simulink model "geometric_control_improved_apf"  (R2025a)
settings: Solver=VariableStepAuto  StartTime=0.0  StopTime=50  RelTol=1e-3
values from neighbouring files (symbols this model uses):
  Ib = diag([1.2416 1.2416 2*1.2416])    [main_geometric_control_improved_apf.m]
  K_a = 1.0    (= 1)    [main_geometric_control_improved_apf.m]
  K_r = 0.5    [main_geometric_control_improved_apf.m]
  K_v = 0.1    [main_geometric_control_improved_apf.m]
  lin_vel_0 = [0; 0; 0]    [main_geometric_control_improved_apf.m]
  mass = 1.2    [main_geometric_control_improved_apf.m]
  obstacles_points = [obstacles_points, points]    [main_geometric_control_improved_apf.m]
  pos_0 = [x0 y0 z0]    [main_geometric_control_improved_apf.m]
  pos_goal = [xf yf zf]    [main_geometric_control_improved_apf.m]
  psif = 0    [main_geometric_control_improved_apf.m]
  rho_0 = 2.0    (= 2)    [main_geometric_control_improved_apf.m]
  Ts = 0.01    [main_geometric_control_improved_apf.m]
  w_bb_0 = [0; 0; 0]    [main_geometric_control_improved_apf.m]
undefined symbols (not defined in the file or in its folder): DiscIntNeverNeededParam
libraries: uavsimlib x3, robotcorelib x2, eeGeneralControl x1
settings Model: Creator=emman  LastModifiedBy=emman

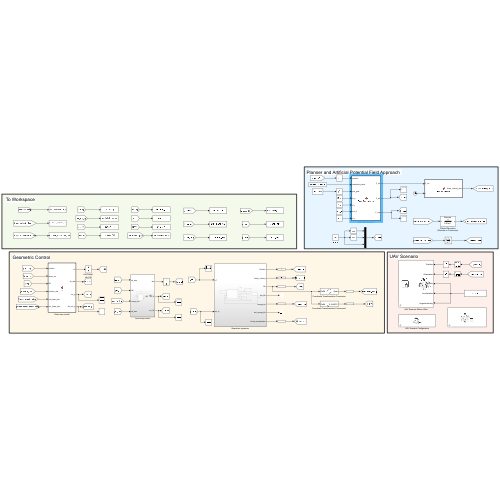
[thumbnail: Simulink's stored preview of the top-level diagram]
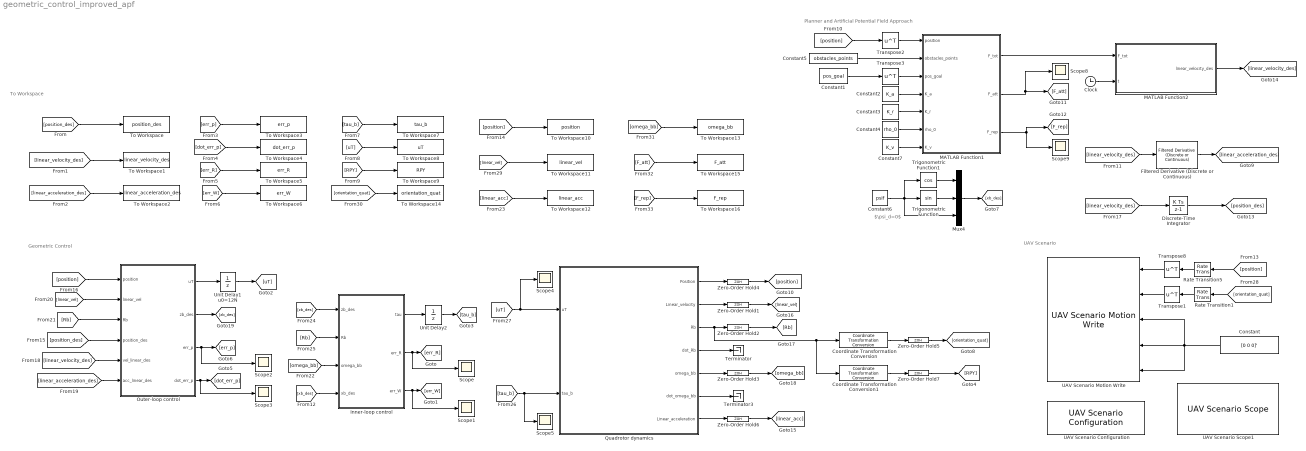
== system geometric_control_improved_apf ==
  note: Planner and Artificial Potential Field Approach
  note: Geometric Control
  note: UAV Scenario
  note: $\psi_d=0$
  note: To Workspace
  Clock : Clock
  Constant : Constant  Value=[0 0 0]'
  Constant1 : Constant  Value=pos_goal
  Constant2 : Constant  Value=K_a
  Constant3 : Constant  Value=K_r
  Constant4 : Constant  Value=rho_0
  Constant5 : Constant  Value=obstacles_points
  Constant6 : Constant  Value=psif
  Constant7 : Constant  Value=K_v
  Coordinate Transformation Conversion : robotcorelib/Coordinate Transformation Conversion  InputRepresentation=Rotation Matrix  InputEulerSequence=ZYX  ShowTrVecInputPort=on  OutputRepresentation=Quaternion  OutputEulerSequence=ZYX  ShowTrVecOutputPort=on  SimulateUsing=Interpreted execution
  Coordinate Transformation Conversion1 : robotcorelib/Coordinate Transformation Conversion  InputRepresentation=Rotation Matrix  InputEulerSequence=ZYX  ShowTrVecInputPort=on  OutputRepresentation=Euler Angles  OutputEulerSequence=ZYX  ShowTrVecOutputPort=on  SimulateUsing=Interpreted execution
  Discrete-Time Integrator : DiscreteIntegrator  InitialCondition=pos_0  SampleTime=Ts  ICPrevOutput=DiscIntNeverNeededParam  ICPrevScaledInput=DiscIntNeverNeededParam
  Filtered Derivative (Discrete or Continuous) : eeGeneralControl/Filtered Derivative (Discrete or Continuous)  K=1  T=Ts  B=inf  A=-inf  minRatio=10  init_option=Inherited from block input  x0=0  Ts=-1
      settings: LibrarySourceBlock=|
      | ee_sl_lib/General Control/Filtered Derivative
      | (Discrete or Continuous)
  Inner-loop control : Subsystem
  MATLAB Function1 : MATLAB Function  TreatAsAtomicUnit=on
  MATLAB Function2 : MATLAB Function  TreatAsAtomicUnit=on
  Mux4 : Mux  Inputs=3
  Outer-loop control : MATLAB Function  TreatAsAtomicUnit=on
  Quadrotor dynamics : Subsystem
  Rate Transition1 : RateTransition  OutPortSampleTime=Ts
  Rate Transition5 : RateTransition  OutPortSampleTime=Ts
  Scope{,1..5,8..9} (8 alike) : Scope
      Scope settings: ActiveDisplayYMinimum=-3.1E-6  ActiveDisplayYMaximum=3.1E-6
      Scope1 settings: ActiveDisplayYMinimum=-1.2E-5  ActiveDisplayYMaximum=1.2E-5
      Scope2 settings: ActiveDisplayYMinimum=-1E-5  ActiveDisplayYMaximum=2E-6  DataLoggingVariableName=ScopeData6
      Scope3 settings: ActiveDisplayYMinimum=-0.00022  ActiveDisplayYMaximum=5E-5  DataLoggingVariableName=ScopeData3
      Scope4 settings: ActiveDisplayYMinimum=11.66748  ActiveDisplayYMaximum=12.03695  DataLoggingVariableName=ScopeData4
      Scope5 settings: ActiveDisplayYMinimum=-0.02035  ActiveDisplayYMaximum=0.02035  DataLoggingVariableName=ScopeData5
      Scope8 settings: ActiveDisplayYMinimum=-10.489441161556352  ActiveDisplayYMaximum=10.433654100091561  DataLoggingVariableName=ScopeData8
      Scope9 settings: ActiveDisplayYMinimum=-1  ActiveDisplayYMaximum=1  DataLoggingVariableName=ScopeData9
  Terminator : Terminator
  Terminator3 : Terminator
  To Workspace : ToWorkspace  VariableName=position_des  SaveFormat=Timeseries  SampleTime=-1
  To Workspace1 : ToWorkspace  VariableName=linear_velocity_des  SaveFormat=Timeseries  SampleTime=-1
  To Workspace10 : ToWorkspace  VariableName=position  SaveFormat=Timeseries  SampleTime=-1
  To Workspace11 : ToWorkspace  VariableName=linear_vel  SaveFormat=Timeseries  SampleTime=-1
  To Workspace12 : ToWorkspace  VariableName=linear_acc  SaveFormat=Timeseries  SampleTime=-1
  To Workspace13 : ToWorkspace  VariableName=omega_bb  SaveFormat=Timeseries  SampleTime=-1
  To Workspace14 : ToWorkspace  VariableName=orientation_quat  SaveFormat=Timeseries  SampleTime=-1
  To Workspace15 : ToWorkspace  VariableName=F_att  SaveFormat=Timeseries  SampleTime=-1
  To Workspace16 : ToWorkspace  VariableName=F_rep  SaveFormat=Timeseries  SampleTime=-1
  To Workspace2 : ToWorkspace  VariableName=linear_acceleration_des  SaveFormat=Timeseries  SampleTime=-1
  To Workspace3 : ToWorkspace  VariableName=err_p  SaveFormat=Timeseries  SampleTime=-1
  To Workspace4 : ToWorkspace  VariableName=dot_err_p  SaveFormat=Timeseries  SampleTime=-1
  To Workspace5 : ToWorkspace  VariableName=err_R  SaveFormat=Timeseries  SampleTime=-1
  To Workspace6 : ToWorkspace  VariableName=err_W  SaveFormat=Timeseries  SampleTime=-1
  To Workspace7 : ToWorkspace  VariableName=tau_b  SaveFormat=Timeseries  SampleTime=-1
  To Workspace8 : ToWorkspace  VariableName=uT  SaveFormat=Timeseries  SampleTime=-1
  To Workspace9 : ToWorkspace  VariableName=RPY  SaveFormat=Timeseries  SampleTime=-1
  Transpose{1..3,8} (4 alike) : Math  Operator=transpose
  Trigonometric Function : Trigonometry
  Trigonometric Function1 : Trigonometry  Operator=cos
  UAV Scenario Configuration : uavsimlib/UAV Scenario Configuration  Priority=-1  UAVScenarioObject=Scenario  SampleTime=Ts  UpdateParam=false  SensorMotionBusName='SensorMotionBus'  PlatformMotionBusName='PlatformMotionBus'  ScenarioMotionBusName='ScenarioMotionBus'  ScenarioMotionSignalName='ScenarioMotions'
  UAV Scenario Motion Write : uavsimlib/UAV Scenario Motion Write  Priority=0  PlatName='UAV'  ReferenceFrame=NED
  UAV Scenario Scope1 : uavsimlib/UAV Scenario Scope  Priority=1  SensorNameTable={}  SampleTime=Ts
  Unit Delay1 u0=12N : UnitDelay  InitialCondition=12  SampleTime=Ts
  Unit Delay2 : UnitDelay  InitialCondition=[0 0 0]  SampleTime=Ts
  Zero-Order Hold{1..7} (7 alike) : ZeroOrderHold  SampleTime=Ts
  wires:
  [linear_velocity_des] -> To Workspace1/1
  Zero-Order Hold3/1 -> [omega_bb]
  [tau_b] -> To Workspace7/1
  [err_R] -> To Workspace5/1
  Coordinate Transformation Conversion1/1 -> Zero-Order Hold7/1
  Coordinate Transformation Conversion/1 -> Zero-Order Hold5/1
  [position_des] -> To Workspace/1
  Quadrotor dynamics/3(Rb) -> Zero-Order Hold2/1, Coordinate Transformation Conversion1/1, Coordinate Transformation Conversion/1
  [err_W] -> To Workspace6/1
  Quadrotor dynamics/6(dot_omega_bb) -> Terminator3/1
  Outer-loop control/3(err_p) -> [err_p], Scope2/1
  Quadrotor dynamics/5(omega_bb) -> Zero-Order Hold3/1
  Outer-loop control/4(dot_err_p) -> [dot_err_p], Scope3/1
  [linear_acceleration_des] -> To Workspace2/1
  Quadrotor dynamics/2(Linear_velocity) -> Zero-Order Hold1/1
  Outer-loop control/1(uT) -> Unit Delay1 u0=12N/1
  Inner-loop control/2(err_R) -> [err_R], Scope/1
  Inner-loop control/3(err_W) -> Scope1/1, [err_W]
  Quadrotor dynamics/4(dot_Rb) -> Terminator/1
  [dot_err_p] -> To Workspace4/1
  [uT] -> To Workspace8/1
  [RPY] -> To Workspace9/1
  Inner-loop control/1(tau) -> Unit Delay2/1
  [err_p] -> To Workspace3/1
  Quadrotor dynamics/1(Position) -> Zero-Order Hold4/1
  Constant2/1 -> MATLAB Function1/4(K_a)
  Constant3/1 -> MATLAB Function1/5(K_r)
  Constant4/1 -> MATLAB Function1/6(rho_0)
  MATLAB Function1/1(F_tot) -> MATLAB Function2/1(F_tot)
  Clock/1 -> MATLAB Function2/2(t)
  MATLAB Function1/2(F_att) -> Scope8/1, [F_att]
  Trigonometric Function1/1 -> Mux4/1
  Mux4/1 -> [xb_des]
  Constant6/1 -> Mux4/3, Trigonometric Function/1, Trigonometric Function1/1
  Trigonometric Function/1 -> Mux4/2
  MATLAB Function2/1(linear_velocity_des) -> [linear_velocity_des]
  [linear_velocity_des] -> Filtered Derivative (Discrete or Continuous)/1
  Filtered Derivative (Discrete or Continuous)/1 -> [linear_acceleration_des]
  [xb_des] -> Inner-loop control/4(xb_des)
  [linear_velocity_des] -> Discrete-Time Integrator/1
  Zero-Order Hold1/1 -> [linear_vel]
  Zero-Order Hold2/1 -> [Rb]
  Zero-Order Hold4/1 -> [position]
  Constant/1 -> UAV Scenario Motion Write/5, UAV Scenario Motion Write/3, UAV Scenario Motion Write/4
  Discrete-Time Integrator/1 -> [position_des]
  Constant5/1 -> MATLAB Function1/2(obstacles_points)
  [position_des] -> Outer-loop control/4(position_des)
  [linear_velocity_des] -> Outer-loop control/5(vel_linear_des)
  [linear_acceleration_des] -> Outer-loop control/6(acc_linear_des)
  Rate Transition5/1 -> Transpose8/1
  [position] -> Rate Transition5/1
  Zero-Order Hold5/1 -> [orientation_quat]
  Quadrotor dynamics/7(Linear_acceleration) -> Zero-Order Hold6/1
  Zero-Order Hold6/1 -> [linear_acc]
  Zero-Order Hold7/1 -> [RPY]
  Outer-loop control/2(zb_des) -> [zb_des]
  [zb_des] -> Inner-loop control/1(zb_des)
  [omega_bb] -> Inner-loop control/3(omega_bb)
  [Rb] -> Inner-loop control/2(Rb)
  Unit Delay2/1 -> [tau_b]
  [tau_b] -> Scope5/1, Quadrotor dynamics/2(tau_b)
  Unit Delay1 u0=12N/1 -> [uT]
  [uT] -> Scope4/1, Quadrotor dynamics/1(uT)
  [position] -> Outer-loop control/1(position)
  [linear_vel] -> Outer-loop control/2(linear_vel)
  [Rb] -> Outer-loop control/3(Rb)
  Transpose8/1 -> UAV Scenario Motion Write/1
  Rate Transition1/1 -> Transpose1/1
  Transpose1/1 -> UAV Scenario Motion Write/2
  [orientation_quat] -> Rate Transition1/1
  [position] -> To Workspace10/1
  [linear_acc] -> To Workspace12/1
  [linear_vel] -> To Workspace11/1
  [omega_bb] -> To Workspace13/1
  [orientation_quat] -> To Workspace14/1
  [F_rep] -> To Workspace16/1
  [F_att] -> To Workspace15/1
  [position] -> Transpose2/1
  Transpose2/1 -> MATLAB Function1/1(position)
  Constant1/1 -> Transpose3/1
  MATLAB Function1/3(F_rep) -> Scope9/1, [F_rep]
  Transpose3/1 -> MATLAB Function1/3(pos_goal)
  Constant7/1 -> MATLAB Function1/7(K_v)

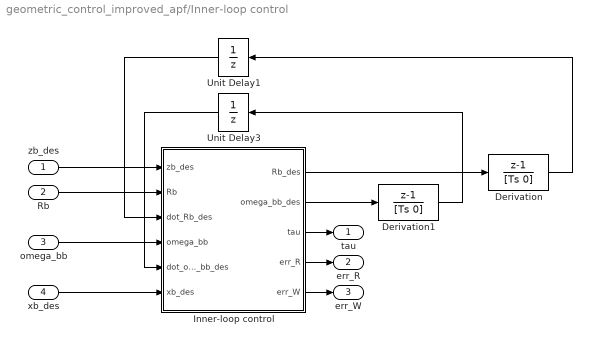
== system geometric_control_improved_apf/Inner-loop control ==
  zb_des : Inport
  Rb : Inport  Port=2
  omega_bb : Inport  Port=3
  xb_des : Inport  Port=4
  Derivation : DiscreteTransferFcn  Numerator=[1 -1]  Denominator=[Ts 0]  InitialStates=[1 0 0;0 1 0;0 0 1]  SampleTime=Ts
  Derivation1 : DiscreteTransferFcn  Numerator=[1 -1]  Denominator=[Ts 0]  InitialStates=[0 0 0]  SampleTime=Ts
  Inner-loop control : MATLAB Function  TreatAsAtomicUnit=on
  Unit Delay1 : UnitDelay  InitialCondition=eye(3)  SampleTime=Ts
  Unit Delay3 : UnitDelay  InitialCondition=[0 0 0]  SampleTime=Ts
  tau : Outport
  err_R : Outport  Port=2
  err_W : Outport  Port=3
  wires:
  xb_des/1 -> Inner-loop control/6(xb_des)
  Inner-loop control/4(err_R) -> err_R/1
  Rb/1 -> Inner-loop control/2(Rb)
  Inner-loop control/3(tau) -> tau/1
  Unit Delay1/1 -> Inner-loop control/3(dot_Rb_des)
  Derivation1/1 -> Unit Delay3/1
  Inner-loop control/5(err_W) -> err_W/1
  Unit Delay3/1 -> Inner-loop control/5(dot_omega_bb_des)
  Derivation/1 -> Unit Delay1/1
  zb_des/1 -> Inner-loop control/1(zb_des)
  omega_bb/1 -> Inner-loop control/4(omega_bb)
  Inner-loop control/1(Rb_des) -> Derivation/1
  Inner-loop control/2(omega_bb_des) -> Derivation1/1

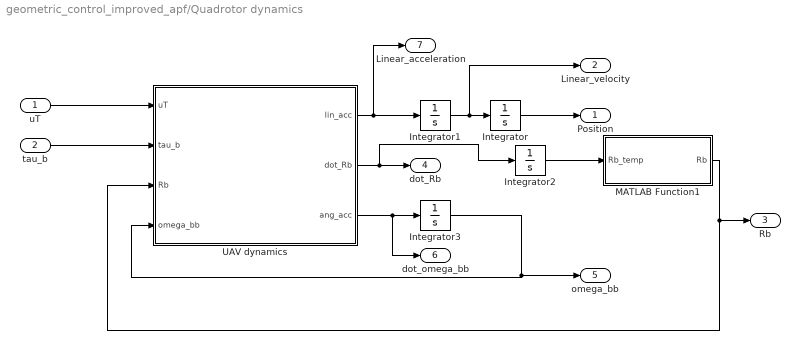
== system geometric_control_improved_apf/Quadrotor dynamics ==
  uT : Inport
  tau_b : Inport  Port=2
  Integrator : Integrator  InitialCondition=pos_0
  Integrator1 : Integrator  InitialCondition=lin_vel_0
  Integrator2 : Integrator  InitialCondition=[1 0 0; 0 1 0;0 0 1]
  Integrator3 : Integrator  InitialCondition=w_bb_0
  MATLAB Function1 : MATLAB Function  TreatAsAtomicUnit=on
  UAV dynamics : MATLAB Function  TreatAsAtomicUnit=on
  Position : Outport
  Linear_velocity : Outport  Port=2
  Rb : Outport  Port=3
  dot_Rb : Outport  Port=4
  omega_bb : Outport  Port=5
  dot_omega_bb : Outport  Port=6
  Linear_acceleration : Outport  Port=7
  wires:
  tau_b/1 -> UAV dynamics/2(tau_b)
  Integrator/1 -> Position/1
  UAV dynamics/3(ang_acc) -> dot_omega_bb/1, Integrator3/1
  UAV dynamics/1(lin_acc) -> Linear_acceleration/1, Integrator1/1
  uT/1 -> UAV dynamics/1(uT)
  Integrator1/1 -> Linear_velocity/1, Integrator/1
  Integrator3/1 -> UAV dynamics/4(omega_bb), omega_bb/1
  UAV dynamics/2(dot_Rb) -> Integrator2/1, dot_Rb/1
  MATLAB Function1/1(Rb) -> Rb/1, UAV dynamics/3(Rb)
  Integrator2/1 -> MATLAB Function1/1(Rb_temp)

== matlab function geometric_control_improved_apf/Quadrotor dynamics/UAV dynamics ==
  data: uT input size=1; tau_b input size=3; lin_acc output size=3; Rb input size=[3,3]; omega_bb input size=3; dot_Rb output size=[3,3]; ang_acc output size=3; mass parameter size=1; Ib parameter size=[3,3]
function [lin_acc, dot_Rb, ang_acc] = fcn(uT,tau_b,Rb,omega_bb,mass, Ib)

lin_acc = 9.81*[0 0 1]'-(uT/mass)*Rb*[0 0 1]';
dot_Rb = Rb*skew(omega_bb);
ang_acc = inv(Ib)*(-skew(omega_bb)*Ib*omega_bb + tau_b);

end

function S = skew(v)
if(numel(v)~= 1)
S= [0 -v(3) v(2); 
    v(3) 0 -v(1);
    -v(2) v(1) 0];
else
S= zeros(3);
end
end

== matlab function geometric_control_improved_apf/Outer-loop control ==
  data: position input size=3; uT output size=1; linear_vel input size=3; Rb input size=[3,3]; zb_des output size=3; mass parameter size=1; position_des input size=3; vel_linear_des input size=3; acc_linear_des input size=3; err_p output size=3; dot_err_p output size=3
function [uT, zb_des, err_p, dot_err_p] = fcn(position, linear_vel, Rb, mass, ...
    position_des, vel_linear_des, acc_linear_des)

%% WRITE HERE THE OUTER-LOOP CONTROL
% position: linear position measure
% linear_vel: linear velocity measure
% Rb: current rotation matrix
% mass: mass of the UAV
% positon_des: desired linear position from the planner
% vel_linear_des: desired linear velocity from the planner
% acc_linear_des: desired linear acceleration from the planner
% ---
% uT: commanded total thrust
% zb_des: desired z-axis of the body frame
% err_p: position error
% dot_err_p: time derivative of the positon error

% Parameters
e3 = [0 0 1]';
g = 9.81;   %Gravity Acceleration

% Errors Computation
err_p = position - position_des;
dot_err_p = linear_vel - vel_linear_des;

% Gains
%K_P = diag([100,100,200]);
%K_V = diag([1,1,20]);

K_P = diag([30,30,60]);
K_V = diag([4,4,20]);

% Commanded Total Thrust 
uT = -(-K_P*err_p - K_V*dot_err_p - mass*g*e3 + mass*acc_linear_des)'*Rb*e3;

% Desired z-axis of the Body Frame
zb_des = -(-K_P*err_p - K_V*dot_err_p -mass*g*e3 + mass*acc_linear_des)/(norm(-K_P*err_p - K_V*dot_err_p -mass*g*e3 + mass*acc_linear_des));

== matlab function geometric_control_improved_apf/Inner-loop control/Inner-loop control ==
  data: Rb_des output size=[3,3]; omega_bb_des output size=3; tau output size=3; zb_des input size=3; Rb input size=[3,3]; dot_Rb_des input size=[3,3]; omega_bb input size=3; dot_omega_bb_des input size=3; xb_des input size=3; Ib parameter size=[3,3]; err_R output size=3; err_W output size=3
function [Rb_des,omega_bb_des,tau,err_R,err_W] = fcn(zb_des,Rb,dot_Rb_des,omega_bb,dot_omega_bb_des,xb_des,Ib)

%% WRITE HERE THE INNER-LOOP CONTROL
% zb_des: desired z-axis of the body frame
% Rb: current rotation matrix
% dot_Rb_des: time-derivative of the desired rotation matrix
% omega_bb: current angular velocity expressed in the body frame
% dot_omega_bb_des: desired angular acceleration expressed in the body
% frame
% xb_des: desired x-axis of the body frame from the planner
% Ib: inertia matrix of the UAV with respect to the body frame
% ---
% Rb_des: desired rotation matrix
% omega_bb_des: desired angular velocity expressed in the body frame (given
% below as a hint)
% tau: commanded control torque
% err_R: rotational error in SO(3)
% err_W: angular velocity error in SO(3)

% Desired Rotational Matrix Computation
yb_des = (skew(zb_des)*xb_des/norm(skew(zb_des)*xb_des));
Rb_des = [skew(yb_des)*zb_des, yb_des, zb_des];

% Desired Angular Velocity Computation in the Body Frame
omega_bb_des = wedge(Rb_des'*dot_Rb_des);

% Errors Computation
err_R = 1/2*wedge(Rb_des'*Rb - Rb'*Rb_des);
err_W = omega_bb - Rb'*Rb_des*omega_bb_des;

% Gains
%K_R = 100*eye(3);
%K_W = 10*eye(3);
K_R = diag([40,40,80]);
K_W = diag([10,10,20]);

% Commanded Control Torque Computation
tau = -K_R*err_R - K_W*err_W + skew(omega_bb)*Ib*omega_bb - Ib*(skew(omega_bb)*Rb'*Rb_des*omega_bb_des - Rb'*Rb_des*dot_omega_bb_des);



end

function S = skew(v)
if(numel(v)~= 1)
S= [0 -v(3) v(2); 
    v(3) 0 -v(1);
    -v(2) v(1) 0];
else
S= zeros(3);
end
end

function v = wedge(S)
v1 = S(3,2);
v2 = S(1,3);
v3 = S(2,1);
v = [v1 v2 v3]';
end

== matlab function geometric_control_improved_apf/Quadrotor dynamics/MATLAB Function1 ==
  data: Rb_temp input; Rb output
function Rb = fcn(Rb_temp)
    [U,S,V] = svd(Rb_temp);
    sigma = det(U*V');
    S_ = diag([1 1 sigma]);

    Rb = U*S_*V';
end

== matlab function geometric_control_improved_apf/MATLAB Function1 ==
  data: position input; F_tot output; obstacles_points input; pos_goal input; K_a input; K_r input; rho_0 input; F_att output; F_rep output; K_v input
function [F_tot, F_att, F_rep] = ForceComputation(position, obstacles_points, pos_goal, K_a, K_r, rho_0, K_v)
% Computes the Total Force (Attractive + Repulsive) for APF (Artificial Potential Field Algorithm)
%
% Inputs:
%   position         - 1x3 UAV Current Position [x, y, z]
%   obstacles_points - 3xN Matrix: each Column is an Obstacle Point [x; y; z] (Different Frame)
%   pos_goal         - 1x3 Goal Position [x, y, z]
%   K_a              - Attractive Force Gain
%   K_r              - Repulsive Force Gain
%   rho_0            - Limit Distance of th Potential Field Influence.
%   K_v              - Virtual Force Gain
%
% Outputs:
%   F_tot            - 1x3 Total Force
%   F_att            - 1x3 Attractive Force
%   F_rep            - 1x3 Repulsive Force


    %% Attractive Force
    % Vector from Current Position to Goal
    e_pos = pos_goal - position;
    
    if norm(e_pos) < 1
        F_att = K_a * e_pos;
    else
        F_att = K_a * e_pos / norm(e_pos);  % Normalization if too far
    end

    %% Repulsive Force (computed from all obstacle points)
    F_rep = zeros(1, 3);  % Initialize total repulsive force vector

    for i = 1:size(obstacles_points, 2)
        obs_point = obstacles_points(:, i)';  % Extract Obstacles Points [1x3]

        % Compute Distance Vectors (Different Frame between Obstacles and UAV)
        dx = position(1) - obs_point(2);
        dy = position(2) - obs_point(1);
        dz = position(3) - obs_point(3);

        rho = sqrt(dx^2 + dy^2 + dz^2);   % Euclidean Distance 

        
        if rho <= rho_0 && rho > 0
            %Gradient = [dx, dy, dz] / rho;  % Gradient (Unit Vector)
            %Repulsion = K_r * (1/rho - 1/rho_0) / rho^2 * Gradient;
            Repulsion = K_v * K_r * (1 - rho/rho_0) * (e_pos/(rho^3)); % Bigger with respect the previous one and so multiplied by a small value
            F_vir = -K_v/rho;
            F_rep = F_rep + Repulsion + F_vir;  % Total Repulsive Force
        end
    end

    %% Total Force = Attractive Force + Repulsive Force
    F_tot = F_att + F_rep;

    %% Tangential Force (Remove the Virtual Force and use the first Repulsion Term with the Gradient)    
    % if norm(F_tot) <= 0.1 && norm(F_rep)~=0
    %      Gradient = [dx, dy, dz] / rho;
    %      F_tan = cross(Gradient, [0,0,1]);
    %      F_tot = F_tot + F_tan;
    % end
end

== matlab function geometric_control_improved_apf/MATLAB Function2 ==
  settings: updateMethod=DISCRETE
  data: F_tot input; t input; linear_velocity_des output
function linear_velocity_des = FilteredVelocity(F_tot, t)
%   This Function apply an Exponential Moving Average Filter to input Total Force Vector
%   It returns the filtered Velocity Vector based on the Input Force Vector F_tot
%   and the Current Time t (for alpha).
%
%   Inputs:
%       F_tot - 1x3 Vector, Total Force Input (from APF Algorithm)
%       t     - Scalar, Current Time (seconds) to compute alpha
%
%   Output:
%       linear_velocity_des - 1x3 Vector, Filtered (Desired) Velocity

% Explanation:
%   In Potential Field Methods, the Output Force Vector represents the direction 
%   and magnitude of "pull" or "push" on the UAV.
%   By applying an Exponential Moving Average Filter to this Force, we can
%   generate a Smoother Velocity Command (linear_velocity_des) that avoids abrupt changes.
%
%   This approach assumes a Proportional relationship between Force and Velocity,
%   effectively treating the Filtered Force as a Desired Velocity Signal.

    % Persistent Variable to store Previous Filtered Velocity
    persistent linear_vel_prev

    if isempty(linear_vel_prev)
        linear_vel_prev = [0 0 0]; % Initialize on First Call
    end

    % Calculate Dynamic Smoothing Factor alpha based on time t
    alpha = alphaComputation(t);

    % Apply Exponential Moving Average Filter
    linear_velocity_des = (1 - alpha) * linear_vel_prev + alpha * F_tot;

    % Update Persistent Variable for Next Iteration
    linear_vel_prev = linear_velocity_des;
end


function alpha = alphaComputation(t)
%   This second function computes alpha for EMA filter adapting over time
%   It returns a Smoothing Factor alpha that increases quadratically
%   from a small initial value up to a final cap.

    alpha_initial = 5e-7; % Initial very small alpha
    alpha_final = 0.005;  % Max alpha value
    % Quadratic increase of alpha over time (example)
    alpha = alpha_initial * (100 * t / 2)^2;

    % Clamp alpha between Initial and Final Values
    alpha = max(min(alpha, alpha_final), alpha_initial);
end
